simulink model "DDWMR"  (R2019b)
settings: Solver=FixedStepAuto  StartTime=0.0  StopTime=20  FixedStep=1e-3  MaxStep=1e-2  RelTol=1e-3
values from neighbouring files (symbols this model uses):
  d = 0.1    [Dynamicfcn.m]    (also in Run_this_file_for_DDWMR_model.m; gps.m)
  I = 0.05    [Dynamicfcn.m]    (also in Run_this_file_for_DDWMR_model.m = 0.26903125)
  L = 0.235/2    (= 0.1175)    [Dynamicfcn.m]    (also in Run_this_file_for_DDWMR_model.m; encoder.m)
  m = 10    [Dynamicfcn.m]    (also in Run_this_file_for_DDWMR_model.m = 15)
  q_initial = [theta_0;x_0;y_0]    [Run_this_file_for_DDWMR_model.m]
  r = 0.05    [Dynamicfcn.m]    (also in Run_this_file_for_DDWMR_model.m; encoder.m; robustness_support.m = temp_r(N+1:-1:1))
  R = 1e-3    (= 0.001)    [Run_this_file_for_DDWMR_model.m]
  Ts = 0.01    [Dynamicfcn.m]    (also in Run_this_file_for_DDWMR_model.m; gps.m = 0.001)
  V_initial = [v_0;w_0]    [Run_this_file_for_DDWMR_model.m]
libraries: simulink x3, sharedTrackingLibrary x1
settings Model: Creator=yz19b  LastModifiedBy=yu zheng

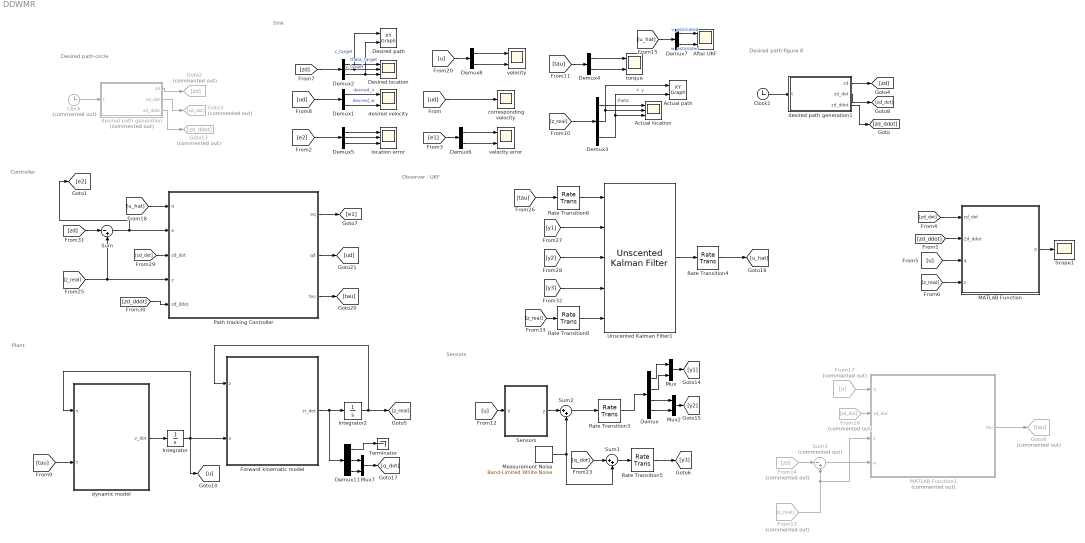
== system DDWMR ==
  note: Desired path-circle
  note: Sink
  note: Controller
  note: Plant
  note: Sensors
  note: Observer - UKF
  note: Desired path-figure 8
  Actual location : Scope  NumInputPorts=3
  Actual path : simulink/Sinks/XY Graph  xmin=-2  xmax=2  ymin=-2  ymax=2  st=-1
  After UKF : Scope  NumInputPorts=2
  Clock : Clock  Commented=on
  Clock1 : Clock
  Demux : Demux
  Demux{1,4,6..8} (5 alike) : Demux  Outputs=2
  Demux{2..3,5,11} (4 alike) : Demux  Outputs=3
  Desired location : Scope  NumInputPorts=3
  "Desired path " : simulink/Sinks/XY Graph  xmin=-2  xmax=2  ymin=-2  ymax=2  st=-1
  Forward kinematic model : MATLAB Function  TreatAsAtomicUnit=on
  From13 : From  Commented=on  GotoTag=z_real
  From14 : From  Commented=on  GotoTag=zd
  From16 : From  Commented=on  GotoTag=zd_dot
  From17 : From  Commented=on  GotoTag=u
  Goto13 : Goto  Commented=on  GotoTag=zd_ddot
  Goto2 : Goto  Commented=on  GotoTag=zd
  Goto3 : Goto  Commented=on  GotoTag=zd_dot
  Goto9 : Goto  Commented=on  GotoTag=tau
  Integrator : Integrator  InitialCondition=V_initial
  Integrator2 : Integrator  InitialCondition=q_initial
  MATLAB Function : MATLAB Function  TreatAsAtomicUnit=on
  MATLAB Function1 : MATLAB Function  Commented=on  TreatAsAtomicUnit=on
  Measurement Noise : simulink/Sources/Band-Limited White Noise  Cov=R*Ts  Ts=Ts  seed=[23341]
  Mux : Mux  Inputs=2
  Mux2 : Mux  Inputs=2
  Mux7 : Mux  Inputs=2
  Path tracking Controller : MATLAB Function  TreatAsAtomicUnit=on
  Rate Transition3 : RateTransition  InitialCondition=[0 0 0 0]  OutPortSampleTime=Ts
  Rate Transition4 : RateTransition  Integrity=off  InitialCondition=1.6  OutPortSampleTime=0
  Rate Transition5 : RateTransition  InitialCondition=[0 0 ]  OutPortSampleTime=Ts
  Rate Transition6 : RateTransition  InitialCondition=[0 0]  OutPortSampleTime=Ts
  Rate Transition8 : RateTransition  InitialCondition=[0 0 0]  OutPortSampleTime=Ts
  Scope1 : Scope
  Sensors : MATLAB Function  TreatAsAtomicUnit=on
  Sum : Sum  Inputs=|-+
  Sum1 : Sum  Inputs=|++
  Sum2 : Sum  Inputs=|++
  Sum3 : Sum  Commented=on  Inputs=|-+
  Terminator : Terminator
  Unscented Kalman Filter1 : sharedTrackingLibrary/Unscented Kalman Filter  StateTransitionFcn=Dynamicfcn  HasAdditiveProcessNoise=Additive  ProcessNoise=diag([1 1])  HasTimeVaryingProcessNoise=off  HasStateTransitionFcnExtraArgument=1  InitialState=[0 0]  InitialStateCovariance=1e-2  Alpha=1e-2  Beta=2  Kappa=0  MeasurementFcn1=gyroscope  HasMeasurementEnablePort1=off  HasAdditiveMeasurementNoise1=Additive  MeasurementNoise1=diag([R R])  HasTimeVaryingMeasurementNoise1=off  HasMeasurementFcnExtraArgument1=0  MeasurementFcn2=encoder  HasMeasurementEnablePort2=off  HasAdditiveMeasurementNoise2=Additive  MeasurementNoise2=diag([R R])  HasTimeVaryingMeasurementNoise2=off  HasMeasurementFcnExtraArgument2=0  MeasurementFcn3=gps  HasMeasurementEnablePort3=off  HasAdditiveMeasurementNoise3=Additive  MeasurementNoise3=diag([R R])  HasTimeVaryingMeasurementNoise3=off  HasMeasurementFcnExtraArgument3=1  MeasurementFcn4=mfcn3  HasMeasurementEnablePort4=off  HasAdditiveMeasurementNoise4=Additive  MeasurementNoise4=R  HasTimeVaryingMeasurementNoise4=off  HasMeasurementFcnExtraArgument4=0  MeasurementFcn5=myMeasurementFcn  HasMeasurementEnablePort5=off  HasAdditiveMeasurementNoise5=Additive  MeasurementNoise5=1  HasTimeVaryingMeasurementNoise5=off  HasMeasurementFcnExtraArgument5=0  EnableMultirate=off  StateTransitionFcnSampleTime=1  MeasurementFcn1SampleTime=1  MeasurementFcn2SampleTime=1  MeasurementFcn3SampleTime=1  MeasurementFcn4SampleTime=1  MeasurementFcn5SampleTime=1  UseCurrentEstimator=on  OutputStateCovariance=off  DataType=double  SampleTime=Ts  NumberOfMeasurements=3
      settings: SourceProductName=Automated Driving Toolbox  SourceProductBaseCode=DR
  corresponding velocity : Scope
  desired path generation : MATLAB Function  Commented=on  TreatAsAtomicUnit=on
  desired path generation1 : MATLAB Function  TreatAsAtomicUnit=on
  desired velocity : Scope  NumInputPorts=2
  dynamic model : MATLAB Function  TreatAsAtomicUnit=on
  location error : Scope  NumInputPorts=3
  torque : Scope  NumInputPorts=2
  velocity : Scope  NumInputPorts=2
  velocity error : Scope  NumInputPorts=2
  wires:
  Clock/1 -> desired path generation/1(t)
  [ud] -> Demux1/1
  Demux1/1 -> desired velocity/1  "desired_v"
  Demux1/2 -> desired velocity/2  "desired_w"
  desired path generation/2(zd_dot) -> Goto3/1
  desired path generation/1(zd) -> Goto2/1
  [zd] -> Demux2/1
  Demux2/1 -> Desired location/1  "theta_target"
  Demux2/2 -> "Desired path "/1, Desired location/2  "x_target"
  Demux2/3 -> "Desired path "/2, Desired location/3  "y_target"
  [tau] -> dynamic model/2(T)
  Forward kinematic model/1(zr_dot) -> Demux11/1, Integrator2/1
  Integrator2/1 -> [z_real], Forward kinematic model/1(z)
  [z_real] -> Demux3/1
  Demux3/3 -> Actual path/2, Actual location/3  "y"
  Demux3/2 -> Actual path/1, Actual location/2  "x"
  Demux3/1 -> Actual location/1  "theta"
  Demux4/2 -> torque/2
  Demux4/1 -> torque/1
  [tau] -> Demux4/1
  [e2] -> Demux5/1
  Demux5/1 -> location error/1
  Demux5/2 -> location error/2
  Demux6/2 -> velocity error/2
  Demux6/1 -> velocity error/1
  [e1] -> Demux6/1
  dynamic model/1(v_dot) -> Integrator/1
  [ud] -> corresponding velocity/1
  [u] -> Sensors/1(V)
  Sensors/1(y) -> Sum2/1
  Sum2/1 -> Rate Transition3/1
  Rate Transition5/1 -> [y3]
  Rate Transition3/1 -> Demux/1
  Demux8/1 -> velocity/1
  Demux8/2 -> velocity/2
  [u] -> Demux8/1
  Demux/1 -> Mux/1
  Demux/2 -> Mux/2
  Demux/3 -> Mux2/1
  Demux/4 -> Mux2/2
  Mux/1 -> [y1]
  Mux2/1 -> [y2]
  [q_dot] -> Sum1/1
  Sum1/1 -> Rate Transition5/1
  Measurement Noise/1 -> Sum1/2, Sum2/2
  Demux7/1 -> After UKF/1  "v_estimated"
  Demux7/2 -> After UKF/2  "w_estimated"
  [u_hat] -> Demux7/1
  Integrator/1 -> Forward kinematic model/2(u), dynamic model/1(v), [u]
  Rate Transition4/1 -> [u_hat]
  [tau] -> Rate Transition6/1
  Unscented Kalman Filter1/1 -> Rate Transition4/1
  Rate Transition6/1 -> Unscented Kalman Filter1/1
  Demux11/2 -> Mux7/1
  Demux11/3 -> Mux7/2
  Mux7/1 -> [q_dot]
  Demux11/1 -> Terminator/1
  [y1] -> Unscented Kalman Filter1/2
  [y2] -> Unscented Kalman Filter1/3
  [y3] -> Unscented Kalman Filter1/4
  [z_real] -> Rate Transition8/1
  Rate Transition8/1 -> Unscented Kalman Filter1/5
  desired path generation1/1(zd) -> [zd]
  desired path generation1/2(zd_dot) -> [zd_dot]
  Clock1/1 -> desired path generation1/1(t)
  desired path generation/3(zd_ddot) -> Goto13/1
  [z_real] -> Sum/2, Path tracking Controller/4(z)
  [zd_dot] -> Path tracking Controller/3(zd_dot)
  [zd_ddot] -> Path tracking Controller/5(zd_ddot)
  [zd] -> Sum/1
  Sum/1 -> [e2], Path tracking Controller/2(e)
  Path tracking Controller/3(tau) -> [tau]
  Path tracking Controller/2(qd) -> [ud]
  desired path generation1/3(zd_ddot) -> [zd_ddot]
  Demux5/3 -> location error/3
  Path tracking Controller/1(eq) -> [e1]
  [z_real] -> MATLAB Function/4(z)
  [zd_ddot] -> MATLAB Function/2(Zd_ddot)
  [zd_dot] -> MATLAB Function/1(zd_dot)
  [u] -> MATLAB Function/3(q)
  MATLAB Function/1(P) -> Scope1/1
  From14/1 -> Sum3/1
  From13/1 -> MATLAB Function1/3(z), Sum3/2
  Sum3/1 -> MATLAB Function1/4(e)
  From16/1 -> MATLAB Function1/2(zd_dot)
  From17/1 -> MATLAB Function1/1(q)
  MATLAB Function1/1(tau) -> Goto9/1
  [u_hat] -> Path tracking Controller/1(q)

== matlab function DDWMR/desired path generation1 ==
  data: t input; zd output; zd_dot output; zd_ddot output
function [zd,zd_dot,zd_ddot] = fcn(t)

a=1;
x = a*cos(t)/(1+sin(t)^2);
y = a*sin(t)*cos(t)/(1+sin(t)^2);
% unit circle (radius = 1; origin: (0,0))
zd = [atan(y./x);              % theta
      a*cos(t)/(1+sin(t)^2);         % x
      a*sin(t)*cos(t)/(1+sin(t)^2)];        % y

zd_dot = [-a*sin(t)*(cos(t)^2+2)/(1+sin(t)^2)^2;
          (a*cos(t)^2-2*a*sin(t)^2)/(1+sin(t)^2)^2];

z1 = (a*sin(t)^2*cos(t)^3-11*a*cos(t)^3+8*a*cos(t))/(1+sin(t)^2)^3;
z2 = -2*a*sin(t)*cos(t)*(3+2*cos(t)^2-sin(t)^2)/(1+sin(t)^2)^3;
zd_ddot = [z1;
           z2];

== matlab function DDWMR/MATLAB Function ==
  data: zd_dot input; P output; Zd_ddot input; q input; z input; m parameter; d parameter; r parameter; L parameter; I parameter
function P = fcn(zd_dot,Zd_ddot,q,z,m, d, r, L, I)

omega = q(2);
% theta = z(1);
x = z(2);
y = z(3);
theta = atan(y/x);


B_inver=-(r/(2*L))*[-L,-1;-L,1];
M=[m,0;
   0,m*d*d+I];
M_temp=[m*d*d+I,0;
         0,m];
M_inver=(1/(m*(m*d*d+I)))*M_temp;
C = [cos(theta), -d*sin(theta);
     sin(theta), d*cos(theta)];
C_inver = (1/d)*[d*cos(theta), d*sin(theta);
                 -sin(theta), cos(theta)];
C_dot = omega*[-sin(theta), -d*cos(theta);
                cos(theta), -d*sin(theta)];
D=[0,-m*d*omega;
    m*d*omega,0];


a1=1;
g_inver = B_inver*M*C_inver;
f = C_dot*q-C*M_inver*D*q-Zd_ddot;
x2 = C*q-zd_dot;
g0 = 1.89;

p =g_inver*(f+a1*x2);
P = norm(p);

== matlab function DDWMR/MATLAB Function1 ==
  data: q input; tau output; zd_dot input; z input; e input; d parameter
function tau = fcn(q,zd_dot,z,e, d)


theta =z(1);
C = [cos(theta), -d*sin(theta);
     sin(theta), d*cos(theta)];
x1 =e(2:3);
x2 = C*q-zd_dot;
a1 =1;


S = x2+a1*x1;


k1 =5000;
k2 =10000;
tau = -k1*S-k2*sign(S);

== matlab function DDWMR/Sensors ==
  data: V input; y output; r parameter; L parameter
function y = fcn(V,r,L)

C=[1,0;
    0,1;
    1/(4*r),L/(4*r);
    1/(4*r),-L/(4*r)];
y=C*V;

== matlab function DDWMR/Path tracking Controller ==
  data: eq output; qd output; q input; tau output; e input; zd_dot input; z input; zd_ddot input; m parameter; d parameter; r parameter; L parameter; I parameter
function [eq,qd,tau] = fcn(q,e,zd_dot,z,zd_ddot,m, d, r, L, I)


kq =15;
ke =15;
ez = e(2:3);
% e_theta = e(1);
theta = z(1);
omega = q(2);

B_inver=-(r/(2*L))*[-L,-1;-L,1];
M=[m,0;
    0,m*d*d+I];
D=[0,-m*d*omega;
    m*d*omega,0];
C = [cos(theta), -d*sin(theta);
     sin(theta), d*cos(theta)];
C_bar_tran = [0, cos(theta), sin(theta);
              1, -d*sin(theta), d*cos(theta)];
C_inver = (1/d)*[d*cos(theta), d*sin(theta);
                 -sin(theta), cos(theta)];
C_inver_dot = (1/d)*[-d*sin(theta)*omega, d*cos(theta)*omega;
                     -cos(theta)*omega, -sin(theta)*omega];


qd = C_inver*(zd_dot-ke*ez);
qd_dot = -ke*(C_inver_dot*ez+q)+C_inver*(zd_ddot+ke*zd_dot+C*C_inver_dot*zd_dot);
u = -kq*(q-qd)+qd_dot-C_bar_tran*e;
tau = B_inver*(M*u+D*q);
eq = q-qd;

== matlab function DDWMR/Forward kinematic model ==
  data: z input; u input; zr_dot output; d parameter; r parameter
function zr_dot = fcn(z,u,d,r)

%% unpacking the state vectors
theta=z(1);

%% unpacking the intput
v=u(1);
omega=u(2);

%% ODE
theta_dot=omega;
x_dot=v*cos(theta)-d*omega*sin(theta);
y_dot=v*sin(theta)+d*omega*cos(theta);
% phir_dot = (v+omega)/r;
% phil_dot = (v-omega)/r;


%% packing the output
zr_dot=[theta_dot;x_dot;y_dot];

== matlab function DDWMR/dynamic model ==
  data: v_dot output; v input; T input; L parameter; r parameter; d parameter; m parameter; I parameter
function v_dot = fcn(v, T,L, r, d, m,I)

%% unpacking intput
omega=v(2);

%% Parameter
M_temp=[m*d*d+I,0;
         0,m];

M_inver=(1/(m*(m*d*d+I)))*M_temp;

D=[0,-m*d*omega;
    m*d*omega,0];

B=(1/r)*[1,1;L,-L];

%% ODE
v_dot=M_inver*(-D*v+B*T);

== matlab function DDWMR/desired path generation ==
  data: t input; zd output; zd_dot output; zd_ddot output
function [zd,zd_dot,zd_ddot] = fcn(t)


% unit circle (radius = 1; origin: (0,0))
zd = [t;
      cos(t);         % x
      sin(t)];        % y

zd_dot = [-sin(t);
          cos(t)];
      
zd_ddot = [-cos(t);
           -sin(t)];
